simulink model "evslx"  (R2025b)
settings: Solver=VariableStepAuto  StartTime=0.0  StopTime=3600  RelTol=1e-3

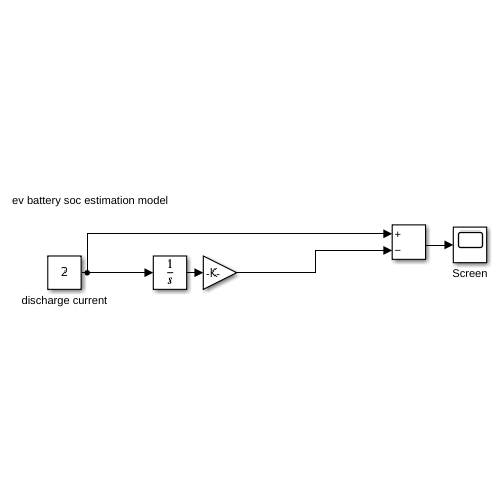
[thumbnail: Simulink's stored preview of the top-level diagram]
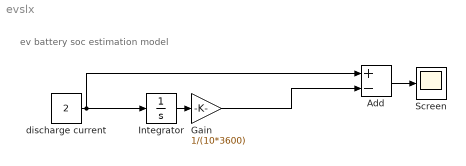
== system evslx ==
  note: ev battery soc estimation model
  Add : Sum  Inputs=+-
  Gain : Gain  Gain=1/(10*3600)
  Integrator : Integrator
  Screen : Scope
      settings: ActiveDisplayYMinimum=1.775  ActiveDisplayYMaximum=2.025
  discharge current : Constant  Value=2
  wires:
  Integrator/1 -> Gain/1
  Gain/1 -> Add/2
  discharge current/1 -> Add/1, Integrator/1
  Add/1 -> Screen/1
